simulink model "sampleModel1705"  (R2023a)
settings: Solver=VariableStepAuto  StartTime=0.0  StopTime=10.0  RelTol=1e-3
libraries: hdlsllib x9, simulink x2
settings Model: Creator=user1  LastModifiedBy=user1

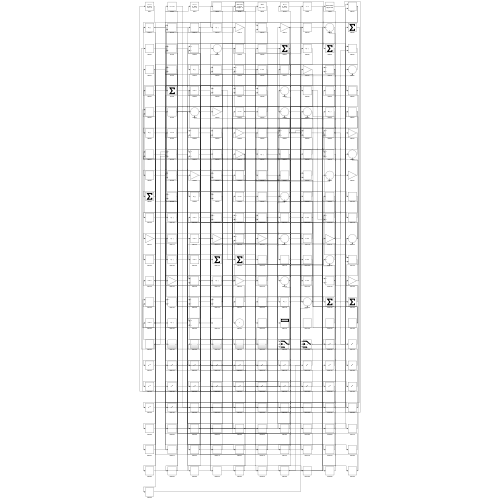
[thumbnail: Simulink's stored preview of the top-level diagram]
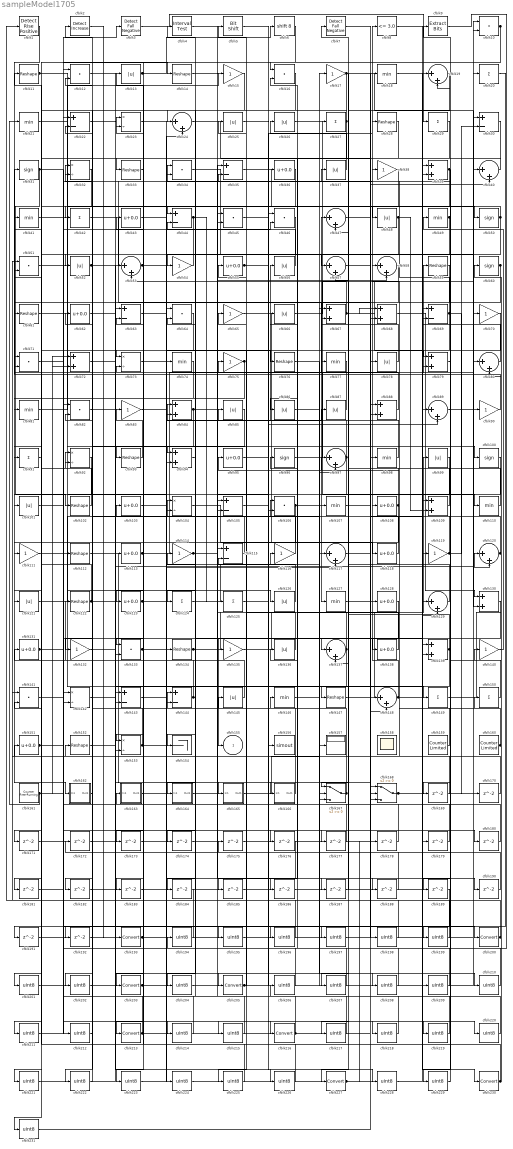
== system sampleModel1705 ==
  cfblk1 : hdlsllib/Logic and Bit Operations/Detect Rise Positive  vinit=0  OutDataTypeStr=boolean
  cfblk{10,12,16,34,45..46,51,64,71,82,106,133,141} (13 alike) : DotProduct  OutDataTypeStr=Inherit: Inherit via internal rule
  cfblk{31,50,60,96,100} (5 alike) : Signum
  cfblk{13,25..26,37,48,52,56,66,78,85..87,99,101,121,126,136,145} (18 alike) : Abs  SaturateOnIntegerOverflow=off
  cfblk{11,14,28,33,59,61,76,93,102,112,122,134,147,152} (14 alike) : Reshape
  cfblk{36,43,55,62,95,103,108,113,118,123,128,131,138,151} (14 alike) : Bias  Bias=0.0  SaturateOnIntegerOverflow=off
  cfblk{23,32,73,92,104,142,153} (7 alike) : Product  Inputs=*/  RndMeth=Zero  SaturateOnIntegerOverflow=on
  cfblk{22,30,35,44,63,69,105,115,143..144} (10 alike) : Sum  Inputs=+-
  cfblk{18,21,41,49,74,77,81,98,107,110,127,146} (12 alike) : MinMax
  cfblk{39,67..68,72,79,84,88,94,109,130,139} (11 alike) : Sum
  cfblk{15,17,38,54,65,70,75,83,90,111,114,116,119,132,135,140} (16 alike) : Gain
  cfblk{19,24,40,47,53,57..58,80,89,97,117,120,129,137,148} (15 alike) : Sum  Inputs=|++
  cfblk{20,27,29,42,91,124..125,149..150} (9 alike) : Sum  Inputs=+
  cfblk154 : Terminator
  cfblk156 : ToWorkspace  VariableName=simout  SaveFormat=Timeseries  SampleTime=-1
  cfblk157 : Display
  cfblk158 : Scope
      settings: Floating=on
  cfblk159 : hdlsllib/Sources/Counter Limited  uplimit=7  tsamp=-1
  cfblk160 : hdlsllib/Sources/Counter Limited  uplimit=7  tsamp=-1
  cfblk161 : hdlsllib/Sources/Counter Free-Running  NumBits=16  tsamp=-1
  cfblk162 : Subsystem
      settings: LibrarySourceBlock=|
      | hdlsllib/Ports &
      | Subsystems/Subsystem
  cfblk163 : Subsystem
      settings: LibrarySourceBlock=|
      | hdlsllib/Ports &
      | Subsystems/Subsystem
  cfblk164 : Subsystem
      settings: LibrarySourceBlock=|
      | hdlsllib/Ports &
      | Subsystems/Subsystem
  cfblk165 : Subsystem
      settings: LibrarySourceBlock=|
      | hdlsllib/Ports &
      | Subsystems/Subsystem
  cfblk166 : Subsystem
      settings: LibrarySourceBlock=|
      | hdlsllib/Ports &
      | Subsystems/Subsystem
  cfblk167 : Switch  SaturateOnIntegerOverflow=off  InputSameDT=off
  cfblk168 : Switch  SaturateOnIntegerOverflow=off  InputSameDT=off
  cfblk{169..192} (24 alike) : Delay  SampleTime=1
  cfblk{193,200,203,205,213,216,227,230} (8 alike) : DataTypeConversion  SaturateOnIntegerOverflow=off  RndMeth=Floor
  cfblk{194..199,201..202,204,206..212,214..215,217..226,228..229,231} (31 alike) : DataTypeConversion  OutDataTypeStr=uint8  SaturateOnIntegerOverflow=off  RndMeth=Floor
  cfblk2 : simulink/Logic and Bit Operations/Detect Increase  vinit=0.0  OutDataTypeStr=boolean
      settings: LibrarySourceBlock=|
      | hdlsllib/Logic and Bit
      | Operations/Detect
      | Increase
  cfblk3 : hdlsllib/Logic and Bit Operations/Detect Fall Negative  vinit=0  OutDataTypeStr=boolean
  cfblk4 : hdlsllib/Logic and Bit Operations/Interval Test  IntervalClosedRight=on  uplimit=0.5  IntervalClosedLeft=on  lowlimit=-0.5  OutDataTypeStr=boolean
  cfblk5 : hdlsllib/Logic and Bit Operations/Bit Shift  mode=Shift Left Logical  N=0
  cfblk6 : ArithShift  BitShiftNumber=8
  cfblk7 : hdlsllib/Logic and Bit Operations/Detect Fall Negative  vinit=0  OutDataTypeStr=boolean
  cfblk8 : hdlsllib/Logic and Bit Operations/Compare To Constant  relop=<=  const=3.0  OutDataTypeStr=boolean
  cfblk9 : simulink/Logic and Bit Operations/Extract Bits  bitsToExtract=Upper half  numBits=8  bitIdxRange=[0 7]  outScalingMode=Preserve fixed-point scaling
      settings: LibrarySourceBlock=|
      | hdlsllib/Logic and Bit
      | Operations/Extract Bits
  cfblk155 : Outport  VectorParamsAs1DForOutWhenUnconnected=off
  wires:
  cfblk41/1 -> cfblk44/1
  cfblk61/1 -> cfblk126/1
  cfblk134/1 -> cfblk8/1, cfblk129/1
  cfblk37/1 -> cfblk26/1
  cfblk68/1 -> cfblk130/1
  cfblk26/1 -> cfblk110/1
  cfblk31/1 -> cfblk102/1, cfblk138/1
  cfblk112/1 -> cfblk165/1(In1)
  cfblk3/1 -> cfblk29/1
  cfblk113/1 -> cfblk59/1, cfblk218/1
  cfblk2/1 -> cfblk193/1
  cfblk87/1 -> cfblk47/1
  cfblk1/1 -> cfblk162/1(In1)
  cfblk35/1 -> cfblk48/1
  cfblk149/1 -> cfblk60/1
  cfblk118/1 -> cfblk44/2
  cfblk148/1 -> cfblk108/1, cfblk129/2
  cfblk59/1 -> cfblk127/1
  cfblk64/1 -> cfblk213/1
  cfblk129/1 -> cfblk103/1
  cfblk98/1 -> cfblk56/1
  cfblk135/1 -> cfblk88/1
  cfblk111/1 -> cfblk149/1
  cfblk88/1 -> cfblk31/1
  cfblk78/1 -> cfblk47/2
  cfblk44/1 -> cfblk54/1, cfblk125/1, cfblk192/1
  cfblk91/1 -> cfblk11/1
  cfblk65/1 -> cfblk118/1
  cfblk97/1 -> cfblk101/1, cfblk5/1
  cfblk140/1 -> cfblk49/1
  cfblk60/1 -> cfblk94/1, cfblk201/1
  cfblk38/1 -> cfblk123/1
  cfblk95/1 -> cfblk156/1
  cfblk114/1 -> cfblk58/2, cfblk84/2
  cfblk119/1 -> cfblk13/1, cfblk30/2
  cfblk90/1 -> cfblk71/1
  cfblk86/1 -> cfblk157/1
  cfblk166/1(Out1) -> cfblk4/1
  cfblk167/1 -> cfblk144/1, cfblk62/1
  cfblk67/1 -> cfblk79/1, cfblk39/1, cfblk53/2, cfblk68/1
  cfblk27/1 -> cfblk24/1, cfblk86/1, cfblk231/1
  cfblk21/1 -> cfblk144/2
  cfblk55/1 -> cfblk28/1, cfblk68/2
  cfblk6/1 -> cfblk16/1
  cfblk32/1 -> cfblk121/1
  cfblk10/1 -> cfblk73/1, cfblk181/1
  cfblk46/1 -> cfblk94/2
  cfblk75/1 -> cfblk81/1, cfblk184/1
  cfblk81/1 -> cfblk15/1
  cfblk15/1 -> cfblk61/1
  cfblk13/1 -> cfblk6/1, cfblk173/1
  cfblk47/1 -> cfblk100/1
  cfblk165/1(Out1) -> cfblk107/1
  cfblk53/1 -> cfblk93/1, cfblk117/2
  cfblk29/1 -> cfblk147/1
  cfblk104/1 -> cfblk128/1
  cfblk116/1 -> cfblk92/1
  cfblk137/1 -> cfblk96/1, cfblk153/2
  cfblk11/1 -> cfblk50/1, cfblk14/1
  cfblk36/1 -> cfblk203/1
  cfblk121/1 -> cfblk17/1
  cfblk23/1 -> cfblk57/1
  cfblk52/1 -> cfblk38/1, cfblk168/3, cfblk214/1
  cfblk145/1 -> cfblk122/1
  cfblk28/1 -> cfblk77/1
  cfblk159/1 -> cfblk104/1
  cfblk122/1 -> cfblk104/2, cfblk71/2
  cfblk42/1 -> cfblk168/2
  cfblk128/1 -> cfblk164/1(In1)
  cfblk147/1 -> cfblk99/1
  cfblk99/1 -> cfblk133/1
  cfblk130/1 -> cfblk155/1
  cfblk70/1 -> cfblk111/1
  cfblk160/1 -> cfblk150/1, cfblk95/1, cfblk84/1
  cfblk151/1 -> cfblk131/1, cfblk3/1, cfblk72/2
  cfblk50/1 -> cfblk42/1, cfblk186/1
  cfblk152/1 -> cfblk133/2
  cfblk39/1 -> cfblk91/1, cfblk34/2, cfblk229/1
  cfblk24/1 -> cfblk88/2
  cfblk150/1 -> cfblk69/1
  cfblk58/1 -> cfblk124/1
  cfblk5/1 -> cfblk46/1
  cfblk89/1 -> cfblk20/1
  cfblk51/1 -> cfblk139/1
  cfblk110/1 -> cfblk85/1
  cfblk125/1 -> cfblk89/2
  cfblk40/1 -> cfblk33/1
  cfblk69/1 -> cfblk35/2, cfblk170/1, cfblk185/1
  cfblk83/1 -> cfblk134/1
  cfblk126/1 -> cfblk55/1
  cfblk72/1 -> cfblk113/1
  cfblk30/1 -> cfblk79/2
  cfblk12/1 -> cfblk216/1
  cfblk109/1 -> cfblk75/1
  cfblk96/1 -> cfblk40/1
  cfblk93/1 -> cfblk83/1
  cfblk45/1 -> cfblk200/1
  cfblk138/1 -> cfblk66/1
  cfblk106/1 -> cfblk97/2, cfblk211/1
  cfblk102/1 -> cfblk51/2
  cfblk82/1 -> cfblk205/1
  cfblk132/1 -> cfblk120/1
  cfblk131/1 -> cfblk112/1, cfblk215/1
  cfblk144/1 -> cfblk114/1, cfblk41/1
  cfblk163/1(Out1) -> cfblk106/1
  cfblk77/1 -> cfblk73/2
  cfblk103/1 -> cfblk87/1
  cfblk101/1 -> cfblk37/1
  cfblk54/1 -> cfblk52/1
  cfblk49/1 -> cfblk183/1, cfblk217/1
  cfblk115/1 -> cfblk23/1
  cfblk117/1 -> cfblk109/1
  cfblk57/1 -> cfblk148/1
  cfblk124/1 -> cfblk27/1
  cfblk48/1 -> cfblk137/1, cfblk109/2, cfblk171/1
  cfblk133/1 -> cfblk24/2, cfblk190/1
  cfblk123/1 -> cfblk166/1(In1), cfblk153/1
  cfblk56/1 -> cfblk34/1
  cfblk17/1 -> cfblk167/1, cfblk90/1, cfblk202/1
  cfblk161/1 -> cfblk21/1, cfblk46/2, cfblk72/1
  cfblk84/1 -> cfblk132/1, cfblk106/2
  cfblk127/1 -> cfblk139/2
  cfblk168/1 -> cfblk69/2, cfblk10/2
  cfblk34/1 -> cfblk130/2
  cfblk66/1 -> cfblk30/1
  cfblk62/1 -> cfblk53/1
  cfblk73/1 -> cfblk76/1
  cfblk19/1 -> cfblk227/1
  cfblk162/1(Out1) -> cfblk32/1
  cfblk92/1 -> cfblk142/2
  cfblk136/1 -> cfblk25/1
  cfblk120/1 -> cfblk97/1, cfblk65/1
  cfblk108/1 -> cfblk154/1, cfblk67/2
  cfblk153/1 -> cfblk92/2, cfblk116/1
  cfblk139/1 -> cfblk7/1, cfblk207/1
  cfblk4/1 -> cfblk135/1
  cfblk80/1 -> cfblk9/1
  cfblk18/1 -> cfblk230/1
  cfblk107/1 -> cfblk40/2
  cfblk79/1 -> cfblk169/1
  cfblk169/1 -> cfblk58/1
  cfblk170/1 -> cfblk51/1
  cfblk171/1 -> cfblk105/2
  cfblk172/1 -> cfblk167/2
  cfblk173/1 -> cfblk168/1
  cfblk94/1 -> cfblk174/1
  cfblk174/1 -> cfblk35/1
  cfblk164/1(Out1) -> cfblk176/1
  cfblk71/1 -> cfblk177/1
  cfblk177/1 -> cfblk142/1
  cfblk178/1 -> cfblk16/2
  cfblk179/1 -> cfblk137/2
  cfblk76/1 -> cfblk180/1
  cfblk180/1 -> cfblk115/2
  cfblk85/1 -> cfblk182/1
  cfblk182/1 -> cfblk148/2
  cfblk183/1 -> cfblk39/2
  cfblk184/1 -> cfblk1/1
  cfblk185/1 -> cfblk67/1
  cfblk186/1 -> cfblk167/3
  cfblk14/1 -> cfblk187/1
  cfblk187/1 -> cfblk57/2
  cfblk25/1 -> cfblk188/1
  cfblk188/1 -> cfblk23/2
  cfblk100/1 -> cfblk189/1
  cfblk190/1 -> cfblk32/2
  cfblk20/1 -> cfblk191/1
  cfblk191/1 -> cfblk89/1
  cfblk192/1 -> cfblk120/2
  cfblk193/1 -> cfblk78/1, cfblk105/1
  cfblk9/1 -> cfblk194/1
  cfblk194/1 -> cfblk2/1
  cfblk175/1 -> cfblk195/1
  cfblk43/1 -> cfblk196/1
  cfblk196/1 -> cfblk175/1
  cfblk141/1 -> cfblk197/1
  cfblk197/1 -> cfblk80/1
  cfblk7/1 -> cfblk198/1
  cfblk198/1 -> cfblk141/1
  cfblk195/1 -> cfblk199/1
  cfblk199/1 -> cfblk141/2
  cfblk200/1 -> cfblk140/1, cfblk43/1
  cfblk201/1 -> cfblk45/1
  cfblk202/1 -> cfblk45/2
  cfblk203/1 -> cfblk117/1, cfblk70/1
  cfblk16/1 -> cfblk204/1
  cfblk204/1 -> cfblk36/1
  cfblk205/1 -> cfblk145/1, cfblk228/1
  cfblk206/1 -> cfblk82/1
  cfblk207/1 -> cfblk82/2
  cfblk146/1 -> cfblk208/1
  cfblk208/1 -> cfblk136/1
  cfblk8/1 -> cfblk209/1
  cfblk209/1 -> cfblk146/1
  cfblk22/1 -> cfblk210/1
  cfblk210/1 -> cfblk10/1
  cfblk211/1 -> cfblk22/1
  cfblk181/1 -> cfblk212/1
  cfblk212/1 -> cfblk22/2
  cfblk213/1 -> cfblk98/1, cfblk152/1
  cfblk214/1 -> cfblk64/1
  cfblk215/1 -> cfblk64/2
  cfblk216/1 -> cfblk206/1, cfblk163/1(In1)
  cfblk217/1 -> cfblk12/1
  cfblk218/1 -> cfblk12/2
  cfblk143/1 -> cfblk219/1
  cfblk219/1 -> cfblk115/1
  cfblk105/1 -> cfblk220/1
  cfblk220/1 -> cfblk143/1
  cfblk189/1 -> cfblk221/1
  cfblk221/1 -> cfblk143/2
  cfblk74/1 -> cfblk222/1
  cfblk222/1 -> cfblk172/1
  cfblk33/1 -> cfblk223/1
  cfblk223/1 -> cfblk74/1
  cfblk63/1 -> cfblk224/1
  cfblk224/1 -> cfblk119/1
  cfblk176/1 -> cfblk225/1
  cfblk225/1 -> cfblk63/1
  cfblk142/1 -> cfblk226/1
  cfblk226/1 -> cfblk63/2
  cfblk227/1 -> cfblk179/1, cfblk178/1
  cfblk228/1 -> cfblk19/1
  cfblk229/1 -> cfblk19/2
  cfblk230/1 -> cfblk80/2, cfblk151/1
  cfblk231/1 -> cfblk18/1

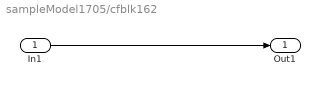
== system sampleModel1705/cfblk162 ==
  In1 : Inport
  Out1 : Outport
  wires:
  In1/1 -> Out1/1

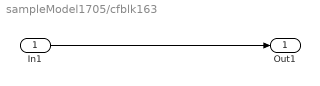
== system sampleModel1705/cfblk163 ==
  In1 : Inport
  Out1 : Outport
  wires:
  In1/1 -> Out1/1

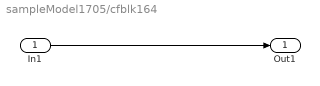
== system sampleModel1705/cfblk164 ==
  In1 : Inport
  Out1 : Outport
  wires:
  In1/1 -> Out1/1

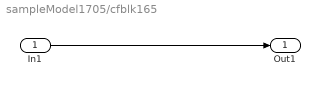
== system sampleModel1705/cfblk165 ==
  In1 : Inport
  Out1 : Outport
  wires:
  In1/1 -> Out1/1

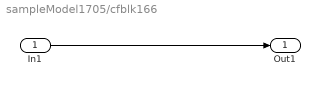
== system sampleModel1705/cfblk166 ==
  In1 : Inport
  Out1 : Outport
  wires:
  In1/1 -> Out1/1
